simulink model "two_link_robot2"  (R2024b)
settings: Solver=VariableStepAuto  StartTime=0.0  StopTime=10.0  RelTol=1e-3
values from neighbouring files (symbols this model uses):
  A = [0 0 1 0 ... (first row only)    [two_link_robot1.m]
  B = [0     0 ... (first row only)    [two_link_robot1.m]
  C = [1 0 0 0 ... (first row only)    [two_link_robot1.m]
  D = [0 0 ... (first row only)    [two_link_robot1.m]
  K = place(A_aug, B_aug, desired_poles)    [two_link_robot1.m]

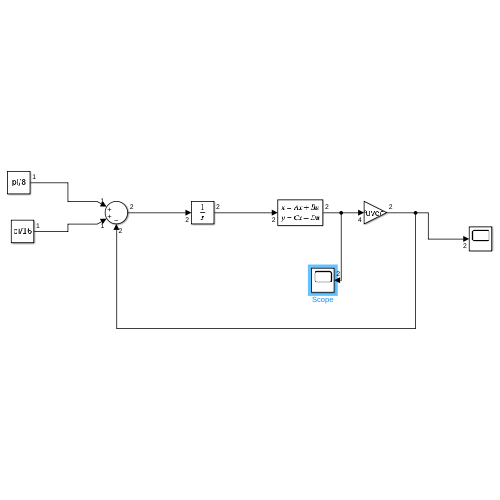
[thumbnail: Simulink's stored preview of the top-level diagram]
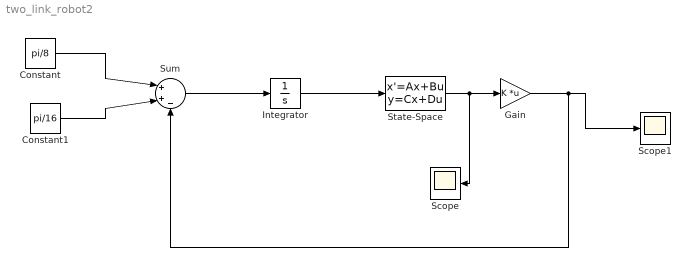
== system two_link_robot2 ==
  Constant : Constant  Value=pi/8
  Constant1 : Constant  Value=pi/16
  Gain : Gain  Gain=K  Multiplication=Matrix(K*u) (u vector)
  Integrator : Integrator  InitialCondition=zeros(2,1)
  Scope : Scope
  Scope1 : Scope
  State-Space : StateSpace  A=A  B=B  C=C  D=D  InitialCondition=zeros(4,1)
  Sum : Sum  Inputs=|++-
  wires:
  Constant/1 -> Sum/1
  Constant1/1 -> Sum/2
  Sum/1 -> Integrator/1
  Integrator/1 -> State-Space/1
  State-Space/1 -> Scope/1, Gain/1
  Gain/1 -> Sum/3, Scope1/1
